simulink model "desafioII_simulink"  (R2016a)
settings: Solver=VariableStepAuto  StartTime=0.0  StopTime=60  RelTol=1e-3
settings Model: Creator=JesseAlves  LastModifiedBy=JesseAlves

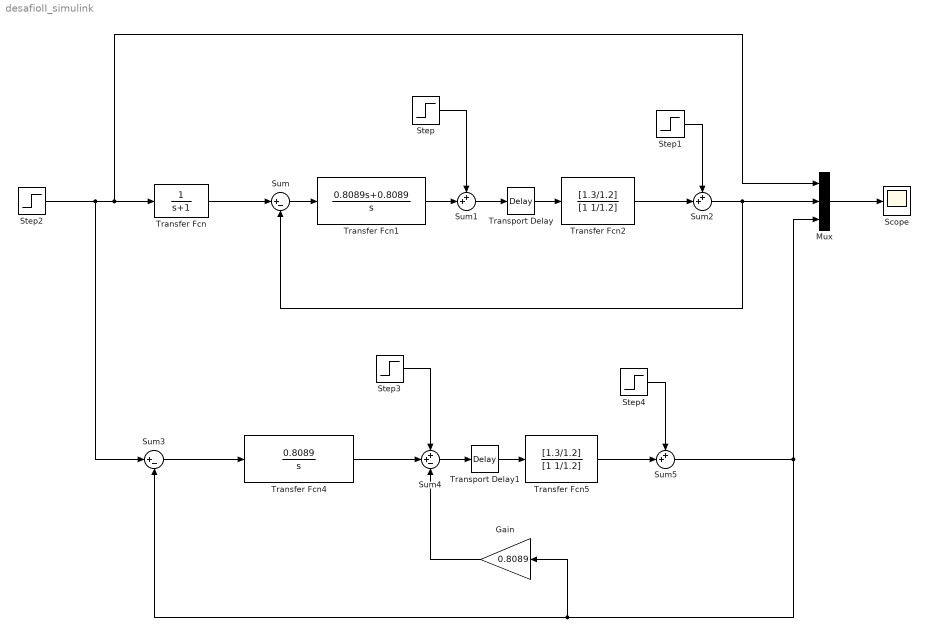
== system desafioII_simulink ==
  Gain : Gain  Gain=0.8089
  Mux : Mux  Inputs=3
  Scope : Scope
  Step : Step  Time=25  After=0.2  SampleTime=0
  Step1 : Step  After=0  SampleTime=0
  Step2 : Step  Time=2  SampleTime=0
  Step3 : Step  Time=25  After=0.2  SampleTime=0
  Step4 : Step  After=0  SampleTime=0
  Sum : Sum  Inputs=|+-
  Sum1 : Sum  Inputs=++|
  Sum2 : Sum  Inputs=++|
  Sum3 : Sum  Inputs=|+-
  Sum4 : Sum  Inputs=++-
  Sum5 : Sum  Inputs=++|
  Transfer Fcn : TransferFcn  Denominator=[1 1]
  Transfer Fcn1 : TransferFcn  Numerator=[0.8089 0.8089]  Denominator=[1 0]
  Transfer Fcn2 : TransferFcn  Numerator=[1.3/1.2]  Denominator=[1 1/1.2]
  Transfer Fcn4 : TransferFcn  Numerator=[0.8089]  Denominator=[1 0]
  Transfer Fcn5 : TransferFcn  Numerator=[1.3/1.2]  Denominator=[1 1/1.2]
  Transport Delay : TransportDelay  DelayTime=0.9
  Transport Delay1 : TransportDelay  DelayTime=0.9
  wires:
  Transfer Fcn/1 -> Sum/1
  Sum/1 -> Transfer Fcn1/1
  Transfer Fcn1/1 -> Sum1/2
  Transfer Fcn2/1 -> Sum2/2
  Step1/1 -> Sum2/1
  Step/1 -> Sum1/1
  Mux/1 -> Scope/1
  Sum2/1 -> Mux/2, Sum/2
  Transport Delay/1 -> Transfer Fcn2/1
  Sum1/1 -> Transport Delay/1
  Step2/1 -> Sum3/1, Transfer Fcn/1, Mux/1
  Sum3/1 -> Transfer Fcn4/1
  Transfer Fcn4/1 -> Sum4/2
  Transfer Fcn5/1 -> Sum5/2
  Step4/1 -> Sum5/1
  Step3/1 -> Sum4/1
  Sum5/1 -> Mux/3, Gain/1, Sum3/2
  Transport Delay1/1 -> Transfer Fcn5/1
  Sum4/1 -> Transport Delay1/1
  Gain/1 -> Sum4/3
